simulink model "verify_create_THB_mdl"  (R2016b)
settings: Solver=VariableStepDiscrete  StartTime=0  StopTime=10  MaxStep=1  RelTol=1e-3  EnableMultiTasking=on
InitFcn:
  | load('DE_TRY2010_13_averageYear')
libraries: simulink x2, carnot x1
settings Model: Creator=drhf  LastModifiedBy=User
settings DataIOCC: SaveFormat=Array  SignalLoggingSaveFormat=ModelDataLogs
settings OptimizationCC: ExpressionDepthLimit=2147483647  LifeSpan=inf
settings DebuggingCC: UnderspecifiedInitializationDetection=Classic  MergeDetectMultiDrivingBlocksExec=none  SolverPrmCheckMsg=warning  FcnCallInpInsideContextMsg=warning  StateNameClashWarn=warning  SFUnexpectedBacktrackingDiag=warning  SFNoUnconditionalDefaultTransitionDiag=warning  SFExecutionAtInitializationDiag=none
settings HardwareCC: ProdBitPerPointer=32  ProdBitPerSizeT=32  ProdBitPerPtrDiffT=32  ProdLargestAtomicFloat=None  ProdIntDivRoundTo=Undefined  ProdEndianess=Unspecified  ProdWordSize=32  ProdHWDeviceType=32-bit Generic
settings ModelReferenceCC: PropagateSignalLabelsOutOfModel=off
settings GRTTargetCC: TargetLangStandard=C89/C90 (ANSI)  GeneratePreprocessorConditionals=Disable all  CombineOutputUpdateFcns=off  GRTInterface=on
settings ConfigComp: CovMetricSettings=dw  CovHtmlReporting=on  CovSaveCumulativeToWorkspaceVar=on  CovSaveSingleToWorkspaceVar=on  CovExternalEMLEnable=off

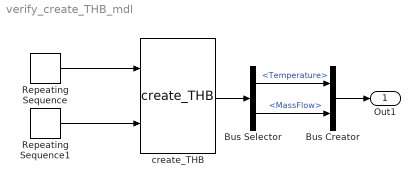
== system verify_create_THB_mdl ==
  Bus Creator : BusCreator  Inputs=2
  Bus Selector : BusSelector  OutputSignals=Temperature,MassFlow
  Repeating Sequence : simulink/Sources/Repeating Sequence  rep_seq_t=[0 5 10]  rep_seq_y=[0 600 0]/3600
  Repeating Sequence1 : simulink/Sources/Repeating Sequence  rep_seq_t=[0 5 10]  rep_seq_y=[20 40 20]
  create_THB : carnot/Source/Simple/create_THB  p=2e5  fluid=Water  mix=0  dia=0.03  mID=No Pressure Drop
  Out1 : Outport
  wires:
  Bus Creator/1 -> Out1/1
  create_THB/1 -> Bus Selector/1
  Repeating Sequence/1 -> create_THB/1
  Repeating Sequence1/1 -> create_THB/2
  Bus Selector/1 -> Bus Creator/1  "<Temperature>"
  Bus Selector/2 -> Bus Creator/2  "<MassFlow>"
